simulink model "PUMA_fuzzy_t1"  (Simulink 8.9)
settings: Solver=ode15s  StartTime=0  StopTime=5  MaxStep=0.02  RelTol=1e-3  EnableMultiTasking=on
undefined symbols (not defined in the file or in its folder): sfunxyz
libraries: aerolibutil x17, simulink x4, fuzblock x3
(part 2 of 3)

== system PUMA_fuzzy_t1/3-Link PUMA Robot-Block /A matrix/a22 generator/I5 ==
  AI5 actual I5 : Constant  Value=0.372
  Sum4 : Sum  Inputs=|++
  UI5 uncertainty added to I5 +- 0.05 max : Constant  Value=UI5
  I5 : Outport
  wires:
  AI5 actual I5/1 -> Sum4/1
  UI5 uncertainty added to I5 +- 0.05 max/1 -> Sum4/2
  Sum4/1 -> I5/1

== system PUMA_fuzzy_t1/3-Link PUMA Robot-Block /A matrix/a22 generator/I6 ==
  AI6 actual I6 : Constant  Value=0.333
  Sum4 : Sum  Inputs=|++
  UI6 uncertainty added to I6 +- 0.05 max : Constant  Value=UI6
  I6 : Outport
  wires:
  AI6 actual I6/1 -> Sum4/1
  UI6 uncertainty added to I6 +- 0.05 max/1 -> Sum4/2
  Sum4/1 -> I6/1

== system PUMA_fuzzy_t1/3-Link PUMA Robot-Block /A matrix/a22 generator/Im2 ==
  AIm2 actual Im2 : Constant  Value=4.71
  Sum4 : Sum  Inputs=|++
  UIm2 uncertainty added to Im2 +- 0.54 max : Constant  Value=UIm2
  Im2 : Outport
  wires:
  AIm2 actual Im2/1 -> Sum4/1
  UIm2 uncertainty added to Im2 +- 0.54 max/1 -> Sum4/2
  Sum4/1 -> Im2/1

== system PUMA_fuzzy_t1/3-Link PUMA Robot-Block /A matrix/a23 generator/I12 ==
  AI12 actual I12 : Constant  Value=-0.011
  Sum4 : Sum  Inputs=|++
  UI12 uncertainty added to I12 +- 0.0011 max : Constant  Value=UI12
  I12 : Outport
  wires:
  AI12 actual I12/1 -> Sum4/1
  UI12 uncertainty added to I12 +- 0.0011 max/1 -> Sum4/2
  Sum4/1 -> I12/1

== system PUMA_fuzzy_t1/3-Link PUMA Robot-Block /A matrix/a23 generator/I15 ==
  AI15 actual I15 : Constant  Value=0.00125
  Sum4 : Sum  Inputs=|++
  UI15 uncertainty added to I15 +- 0.0003 max : Constant  Value=UI15
  I15 : Outport
  wires:
  AI15 actual I15/1 -> Sum4/1
  UI15 uncertainty added to I15 +- 0.0003 max/1 -> Sum4/2
  Sum4/1 -> I15/1

== system PUMA_fuzzy_t1/3-Link PUMA Robot-Block /A matrix/a23 generator/I16 ==
  AI16 actual I16 : Constant  Value=0.00124
  Sum4 : Sum  Inputs=|++
  UI16 uncertainty added to I16 +- 0.0003 max : Constant  Value=UI16
  I16 : Outport
  wires:
  AI16 actual I16/1 -> Sum4/1
  UI16 uncertainty added to I16 +- 0.0003 max/1 -> Sum4/2
  Sum4/1 -> I16/1

== system PUMA_fuzzy_t1/3-Link PUMA Robot-Block /A matrix/a23 generator/I5 ==
  AI5 actual I5 : Constant  Value=0.372
  Sum4 : Sum  Inputs=|++
  UI5 uncertainty added to I5 +- 0.05 max : Constant  Value=UI5
  I5 : Outport
  wires:
  AI5 actual I5/1 -> Sum4/1
  UI5 uncertainty added to I5 +- 0.05 max/1 -> Sum4/2
  Sum4/1 -> I5/1

== system PUMA_fuzzy_t1/3-Link PUMA Robot-Block /A matrix/a23 generator/I6 ==
  AI6 actual I6 : Constant  Value=0.333
  Sum4 : Sum  Inputs=|++
  UI6 uncertainty added to I6 +- 0.05 max : Constant  Value=UI6
  I6 : Outport
  wires:
  AI6 actual I6/1 -> Sum4/1
  UI6 uncertainty added to I6 +- 0.05 max/1 -> Sum4/2
  Sum4/1 -> I6/1

== system PUMA_fuzzy_t1/3-Link PUMA Robot-Block /A matrix/a33 generator/I15 ==
  AI15 actual I15 : Constant  Value=0.00125
  Sum4 : Sum  Inputs=|++
  UI15 uncertainty added to I15 +- 0.0003 max : Constant  Value=UI15
  I15 : Outport
  wires:
  AI15 actual I15/1 -> Sum4/1
  UI15 uncertainty added to I15 +- 0.0003 max/1 -> Sum4/2
  Sum4/1 -> I15/1

== system PUMA_fuzzy_t1/3-Link PUMA Robot-Block /A matrix/a33 generator/I6 ==
  AI6 actual I6 : Constant  Value=0.333
  Sum4 : Sum  Inputs=|++
  UI6 uncertainty added to I6 +- 0.05 max : Constant  Value=UI6
  I6 : Outport
  wires:
  AI6 actual I6/1 -> Sum4/1
  UI6 uncertainty added to I6 +- 0.05 max/1 -> Sum4/2
  Sum4/1 -> I6/1

== system PUMA_fuzzy_t1/3-Link PUMA Robot-Block /A matrix/a33 generator/Im3 ==
  AIm3 actual Im3 : Constant  Value=0.827
  Sum4 : Sum  Inputs=|++
  UIm3 uncertainty added to Im3 +- 0.093 max : Constant  Value=UIm3
  Im3 : Outport
  wires:
  AIm3 actual Im3/1 -> Sum4/1
  UIm3 uncertainty added to Im3 +- 0.093 max/1 -> Sum4/2
  Sum4/1 -> Im3/1

== system PUMA_fuzzy_t1/3-Link PUMA Robot-Block /A matrix/a35 generator/I15 ==
  AI15 actual I15 : Constant  Value=0.00125
  Sum4 : Sum  Inputs=|++
  UI15 uncertainty added to I15 +- 0.0003 max : Constant  Value=UI15
  I15 : Outport
  wires:
  AI15 actual I15/1 -> Sum4/1
  UI15 uncertainty added to I15 +- 0.0003 max/1 -> Sum4/2
  Sum4/1 -> I15/1

== system PUMA_fuzzy_t1/3-Link PUMA Robot-Block /A matrix/a35 generator/I17 ==
  AI17 actual I17 : Constant  Value=0.000642
  Sum4 : Sum  Inputs=|++
  UI17 uncertainty added to I17 +- 0.0003 max : Constant  Value=UI17
  I17 : Outport
  wires:
  AI17 actual I17/1 -> Sum4/1
  UI17 uncertainty added to I17 +- 0.0003 max/1 -> Sum4/2
  Sum4/1 -> I17/1

== system PUMA_fuzzy_t1/3-Link PUMA Robot-Block /A matrix/a44 generator/I14 ==
  AI14 actual I14 : Constant  Value=0.00164
  Sum4 : Sum  Inputs=|++
  UI14 uncertainty added to I14 +- 0.0009 max : Constant  Value=UI14
  I14 : Outport
  wires:
  AI14 actual I14/1 -> Sum4/1
  UI14 uncertainty added to I14 +- 0.0009 max/1 -> Sum4/2
  Sum4/1 -> I14/1

== system PUMA_fuzzy_t1/3-Link PUMA Robot-Block /A matrix/a44 generator/Im4 ==
  AIm4 actual Im4 : Constant  Value=0.2
  Sum4 : Sum  Inputs=|++
  UIm4 uncertainty added to Im4 +- 0.54 max : Constant  Value=UIm4
  Im4 : Outport
  wires:
  AIm4 actual Im4/1 -> Sum4/1
  UIm4 uncertainty added to Im4 +- 0.54 max/1 -> Sum4/2
  Sum4/1 -> Im4/1

== system PUMA_fuzzy_t1/3-Link PUMA Robot-Block /A matrix/a55 generator/I17 ==
  AI17 actual I17 : Constant  Value=0.000642
  Sum4 : Sum  Inputs=|++
  UI17 uncertainty added to I17 +- 0.0003 max : Constant  Value=UI17
  I17 : Outport
  wires:
  AI17 actual I17/1 -> Sum4/1
  UI17 uncertainty added to I17 +- 0.0003 max/1 -> Sum4/2
  Sum4/1 -> I17/1

== system PUMA_fuzzy_t1/3-Link PUMA Robot-Block /A matrix/a55 generator/Im5 ==
  AIm5 actual Im5 : Constant  Value=0.179
  Sum4 : Sum  Inputs=|++
  UIm5 uncertainty added to Im5 +- 0.014 max : Constant  Value=UIm5
  Im5 : Outport
  wires:
  AIm5 actual Im5/1 -> Sum4/1
  UIm5 uncertainty added to Im5 +- 0.014 max/1 -> Sum4/2
  Sum4/1 -> Im5/1

== system PUMA_fuzzy_t1/3-Link PUMA Robot-Block /A matrix/a66 generator/I23 ==
  AI23 actual I23 : Constant  Value=0.00004
  Sum4 : Sum  Inputs=|++
  UI23 uncertainty added to I23 +- 0.00002 max : Constant  Value=UI23
  I23 : Outport
  wires:
  AI23 actual I23/1 -> Sum4/1
  UI23 uncertainty added to I23 +- 0.00002 max/1 -> Sum4/2
  Sum4/1 -> I23/1

== system PUMA_fuzzy_t1/3-Link PUMA Robot-Block /A matrix/a66 generator/Im6 ==
  AIm6 actual Im6 : Constant  Value=0.193
  Sum4 : Sum  Inputs=|++
  UIm6 uncertainty added to Im6 +- 0.54 max : Constant  Value=UIm6
  Im6 : Outport
  wires:
  AIm6 actual Im6/1 -> Sum4/1
  UIm6 uncertainty added to Im6 +- 0.54 max/1 -> Sum4/2
  Sum4/1 -> Im6/1

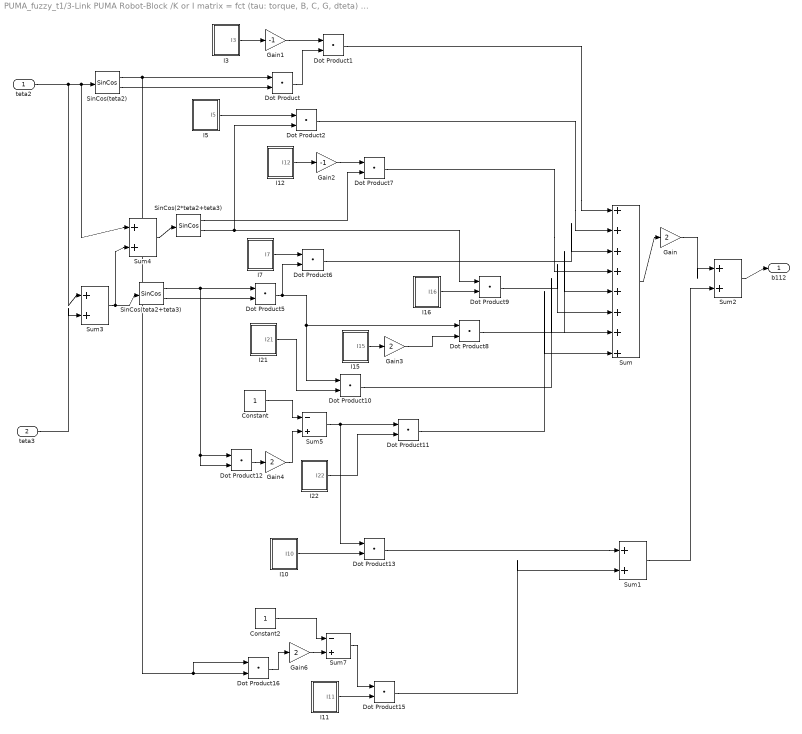
== system PUMA_fuzzy_t1/3-Link PUMA Robot-Block /K or I matrix = fct (tau: torque, B, C, G, dteta) /B matrix/b112 ==
  teta2 : Inport
  teta3 : Inport  Port=2
  Constant : Constant
  Constant2 : Constant
  Dot Product{,1..2,5..13,15..16} (14 alike) : DotProduct  InputSameDT=on  OutDataTypeStr=Inherit: Inherit via internal rule
  Gain{,3..4,6} (4 alike) : Gain  Gain=2
  Gain1 : Gain  Gain=-1
  Gain2 : Gain  Gain=-1
  I10 : Subsystem
  I11 : Subsystem
  I12 : Subsystem
  I15 : Subsystem
  I16 : Subsystem
  I21 : Subsystem
  I22 : Subsystem
  I3 : Subsystem
  I5 : Subsystem
  I7 : Subsystem
  SinCos(2*teta2+teta3) : aerolibutil/SinCos
      settings: SourceProductName=Aerospace Blockset  SourceProductBaseCode=AE
  SinCos(teta2) : aerolibutil/SinCos
      settings: SourceProductName=Aerospace Blockset  SourceProductBaseCode=AE
  SinCos(teta2+teta3) : aerolibutil/SinCos
      settings: SourceProductName=Aerospace Blockset  SourceProductBaseCode=AE
  Sum : Sum  Inputs=|++++++++
  Sum{1..4} (4 alike) : Sum  Inputs=|++
  Sum5 : Sum  Inputs=|-+
  Sum7 : Sum  Inputs=|-+
  b112 : Outport
  wires:
  Sum/1 -> Gain/1
  Gain/1 -> Sum2/1
  Sum1/1 -> Sum2/2
  Sum2/1 -> b112/1
  teta2/1 -> Sum4/1, SinCos(teta2)/1, Sum3/1
  teta3/1 -> Sum3/2
  SinCos(teta2)/1 -> Dot Product/1, Dot Product16/2, Dot Product16/1
  SinCos(teta2)/2 -> Dot Product/2
  Sum3/1 -> SinCos(teta2+teta3)/1, Sum4/2
  I3/1(I3) -> Gain1/1
  Gain1/1 -> Dot Product1/1
  Dot Product/1 -> Dot Product1/2
  Dot Product1/1 -> Sum/1
  Dot Product2/1 -> Sum/2
  I7/1(I7) -> Dot Product6/1
  Dot Product5/1 -> Dot Product6/2, Dot Product8/1, Dot Product10/1
  SinCos(teta2+teta3)/1 -> Dot Product5/1, Dot Product12/1, Dot Product12/2
  SinCos(teta2+teta3)/2 -> Dot Product5/2
  Dot Product6/1 -> Sum/3
  I12/1(I12) -> Gain2/1
  Sum4/1 -> SinCos(2*teta2+teta3)/1
  Gain2/1 -> Dot Product7/1
  SinCos(2*teta2+teta3)/1 -> Dot Product7/2
  Dot Product7/1 -> Sum/4
  I15/1(I15) -> Gain3/1
  Gain3/1 -> Dot Product8/2
  Dot Product8/1 -> Sum/5
  SinCos(2*teta2+teta3)/2 -> Dot Product9/1, Dot Product2/2
  I16/1(I16) -> Dot Product9/2
  Dot Product9/1 -> Sum/6
  I21/1(I21) -> Dot Product10/2
  Dot Product10/1 -> Sum/7
  I22/1(I22) -> Dot Product11/2
  Dot Product12/1 -> Gain4/1
  Constant/1 -> Sum5/1
  Gain4/1 -> Sum5/2
  Sum5/1 -> Dot Product13/1, Dot Product11/1
  Dot Product11/1 -> Sum/8
  I10/1(I10) -> Dot Product13/2
  I11/1(I11) -> Dot Product15/2
  Dot Product16/1 -> Gain6/1
  Constant2/1 -> Sum7/1
  Gain6/1 -> Sum7/2
  Sum7/1 -> Dot Product15/1
  Dot Product13/1 -> Sum1/1
  Dot Product15/1 -> Sum1/2
  I5/1(I5) -> Dot Product2/1

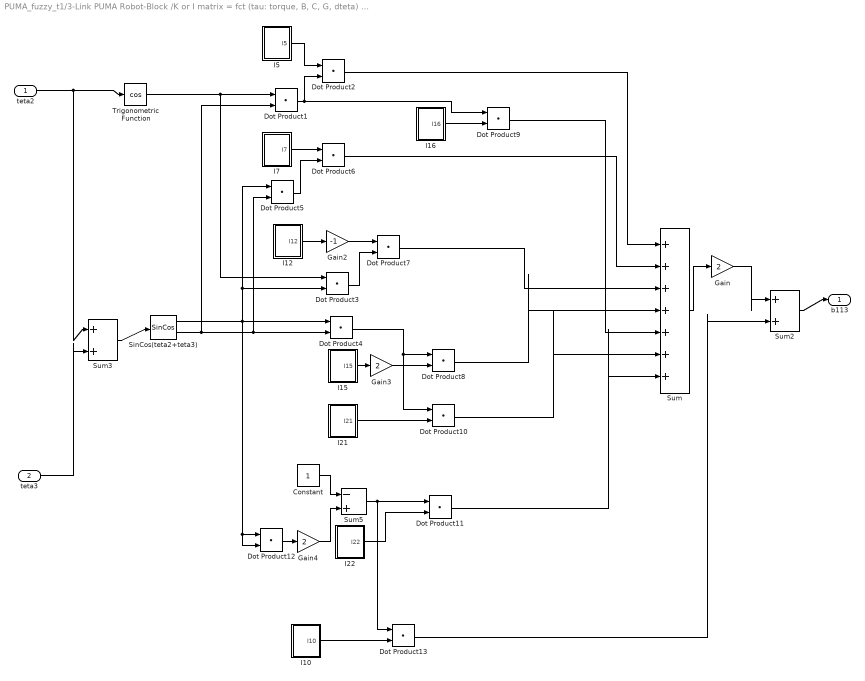
== system PUMA_fuzzy_t1/3-Link PUMA Robot-Block /K or I matrix = fct (tau: torque, B, C, G, dteta) /B matrix/b113 ==
  teta2 : Inport
  teta3 : Inport  Port=2
  Constant : Constant
  Dot Product{1..13} (13 alike) : DotProduct  InputSameDT=on  OutDataTypeStr=Inherit: Inherit via internal rule
  Gain : Gain  Gain=2
  Gain2 : Gain  Gain=-1
  Gain3 : Gain  Gain=2
  Gain4 : Gain  Gain=2
  I10 : Subsystem
  I12 : Subsystem
  I15 : Subsystem
  I16 : Subsystem
  I21 : Subsystem
  I22 : Subsystem
  I5 : Subsystem
  I7 : Subsystem
  SinCos(teta2+teta3) : aerolibutil/SinCos
      settings: SourceProductName=Aerospace Blockset  SourceProductBaseCode=AE
  Sum : Sum  Inputs=|+++++++
  Sum2 : Sum  Inputs=|++
  Sum3 : Sum  Inputs=|++
  Sum5 : Sum  Inputs=|-+
  Trigonometric Function : Trigonometry  Operator=cos
  b113 : Outport
  wires:
  Sum/1 -> Gain/1
  Gain/1 -> Sum2/1
  Sum2/1 -> b113/1
  teta2/1 -> Sum3/1, Trigonometric Function/1
  teta3/1 -> Sum3/2
  Sum3/1 -> SinCos(teta2+teta3)/1
  I7/1(I7) -> Dot Product6/1
  Dot Product5/1 -> Dot Product6/2
  SinCos(teta2+teta3)/1 -> Dot Product5/1, Dot Product3/2, Dot Product4/1, Dot Product12/1, Dot Product12/2
  SinCos(teta2+teta3)/2 -> Dot Product1/2, Dot Product5/2, Dot Product4/2
  I12/1(I12) -> Gain2/1
  Gain2/1 -> Dot Product7/1
  I15/1(I15) -> Gain3/1
  Gain3/1 -> Dot Product8/2
  I16/1(I16) -> Dot Product9/2
  I21/1(I21) -> Dot Product10/2
  I22/1(I22) -> Dot Product11/2
  Dot Product12/1 -> Gain4/1
  Constant/1 -> Sum5/1
  Gain4/1 -> Sum5/2
  Sum5/1 -> Dot Product13/1, Dot Product11/1
  I10/1(I10) -> Dot Product13/2
  I5/1(I5) -> Dot Product2/1
  Dot Product1/1 -> Dot Product2/2, Dot Product9/1
  Trigonometric Function/1 -> Dot Product1/1, Dot Product3/1
  Dot Product3/1 -> Dot Product7/2
  Dot Product4/1 -> Dot Product8/1, Dot Product10/1
  Dot Product13/1 -> Sum2/2
  Dot Product2/1 -> Sum/1
  Dot Product6/1 -> Sum/2
  Dot Product7/1 -> Sum/3
  Dot Product8/1 -> Sum/4
  Dot Product9/1 -> Sum/5
  Dot Product10/1 -> Sum/6
  Dot Product11/1 -> Sum/7

== system PUMA_fuzzy_t1/3-Link PUMA Robot-Block /K or I matrix = fct (tau: torque, B, C, G, dteta) /B matrix/b115 ==
  teta2 : Inport
  teta3 : Inport  Port=2
  Dot Product{,1..5} (6 alike) : DotProduct  InputSameDT=on  OutDataTypeStr=Inherit: Inherit via internal rule
  Gain : Gain  Gain=2
  Gain1 : Gain  Gain=-1
  I15 : Subsystem
  I16 : Subsystem
  I22 : Subsystem
  SinCos(teta2+teta3) : aerolibutil/SinCos
      settings: SourceProductName=Aerospace Blockset  SourceProductBaseCode=AE
  Sum2 : Sum  Inputs=|++++
  Sum3 : Sum  Inputs=|++
  Trigonometric Function : Trigonometry  Operator=cos
  b115 : Outport
  wires:
  teta2/1 -> Sum3/1, Trigonometric Function/1
  teta3/1 -> Sum3/2
  Sum3/1 -> SinCos(teta2+teta3)/1
  SinCos(teta2+teta3)/1 -> Dot Product/1
  SinCos(teta2+teta3)/2 -> Dot Product/2, Dot Product3/1, Dot Product5/1, Dot Product5/2
  Dot Product/1 -> Gain1/1, Dot Product1/1
  I15/1(I15) -> Dot Product1/2
  I16/1(I16) -> Dot Product2/2
  Dot Product3/1 -> Dot Product2/1
  Trigonometric Function/1 -> Dot Product3/2
  Sum2/1 -> Gain/1
  Gain/1 -> b115/1
  I22/1(I22) -> Dot Product4/2
  Dot Product5/1 -> Dot Product4/1
  Gain1/1 -> Sum2/1
  Dot Product1/1 -> Sum2/2
  Dot Product2/1 -> Sum2/3
  Dot Product4/1 -> Sum2/4

== system PUMA_fuzzy_t1/3-Link PUMA Robot-Block /K or I matrix = fct (tau: torque, B, C, G, dteta) /B matrix/b123 ==
  teta2 : Inport
  teta3 : Inport  Port=2
  Dot Product : DotProduct  InputSameDT=on  OutDataTypeStr=Inherit: Inherit via internal rule
  Dot Product1 : DotProduct  InputSameDT=on  OutDataTypeStr=Inherit: Inherit via internal rule
  Dot Product2 : DotProduct  InputSameDT=on  OutDataTypeStr=Inherit: Inherit via internal rule
  Gain : Gain  Gain=2
  Gain1 : Gain  Gain=-1
  I13 : Subsystem
  I18 : Subsystem
  I8 : Subsystem
  SinCos(teta2+teta3) : aerolibutil/SinCos
      settings: SourceProductName=Aerospace Blockset  SourceProductBaseCode=AE
  Sum2 : Sum  Inputs=|+++
  Sum3 : Sum  Inputs=|++
  b123 : Outport
  wires:
  teta2/1 -> Sum3/1
  teta3/1 -> Sum3/2
  Sum3/1 -> SinCos(teta2+teta3)/1
  Dot Product/1 -> Gain1/1
  Sum2/1 -> Gain/1
  Gain/1 -> b123/1
  SinCos(teta2+teta3)/1 -> Dot Product/2, Dot Product2/1
  I8/1(I8) -> Dot Product/1
  SinCos(teta2+teta3)/2 -> Dot Product1/1
  I13/1(I13) -> Dot Product1/2
  I18/1(I18) -> Dot Product2/2
  Gain1/1 -> Sum2/1
  Dot Product1/1 -> Sum2/2
  Dot Product2/1 -> Sum2/3

== system PUMA_fuzzy_t1/3-Link PUMA Robot-Block /K or I matrix = fct (tau: torque, B, C, G, dteta) /B matrix/b214 ==
  teta2 : Inport
  teta3 : Inport  Port=2
  Dot Product1 : DotProduct  InputSameDT=on  OutDataTypeStr=Inherit: Inherit via internal rule
  Dot Product2 : DotProduct  InputSameDT=on  OutDataTypeStr=Inherit: Inherit via internal rule
  Dot Product3 : DotProduct  InputSameDT=on  OutDataTypeStr=Inherit: Inherit via internal rule
  I14 : Subsystem
  I19 : Subsystem
  I20 : Subsystem
  Sum2 : Sum  Inputs=|+++
  Sum3 : Sum  Inputs=|++
  sin(teta2+teta3) : Trigonometry
  b214 : Outport
  wires:
  teta2/1 -> Sum3/1
  teta3/1 -> Sum3/2
  Sum3/1 -> sin(teta2+teta3)/1
  Sum2/1 -> b214/1
  I14/1(I14) -> Dot Product3/1
  sin(teta2+teta3)/1 -> Dot Product3/2, Dot Product1/1, Dot Product2/1
  I19/1(I19) -> Dot Product1/2
  I20/1(I20) -> Dot Product2/2
  Dot Product3/1 -> Sum2/1
  Dot Product1/1 -> Sum2/2
  Dot Product2/1 -> Sum2/3

== system PUMA_fuzzy_t1/3-Link PUMA Robot-Block /K or I matrix = fct (tau: torque, B, C, G, dteta) /B matrix/b223 ==
  teta3 : Inport
  Dot Product1 : DotProduct  InputSameDT=on  OutDataTypeStr=Inherit: Inherit via internal rule
  Dot Product2 : DotProduct  InputSameDT=on  OutDataTypeStr=Inherit: Inherit via internal rule
  Dot Product3 : DotProduct  InputSameDT=on  OutDataTypeStr=Inherit: Inherit via internal rule
  Gain : Gain  Gain=2
  I12 : Subsystem
  I16 : Subsystem
  I5 : Subsystem
  SinCos(teta2+teta3) : aerolibutil/SinCos
      settings: SourceProductName=Aerospace Blockset  SourceProductBaseCode=AE
  Sum2 : Sum  Inputs=|-++
  b223 : Outport
  wires:
  teta3/1 -> SinCos(teta2+teta3)/1
  Dot Product3/1 -> Sum2/1
  Dot Product1/1 -> Sum2/2
  Dot Product2/1 -> Sum2/3
  Sum2/1 -> Gain/1
  Gain/1 -> b223/1
  I12/1(I12) -> Dot Product3/1
  I5/1(I5) -> Dot Product1/2
  I16/1(I16) -> Dot Product2/2
  SinCos(teta2+teta3)/2 -> Dot Product2/1, Dot Product1/1
  SinCos(teta2+teta3)/1 -> Dot Product3/2

== system PUMA_fuzzy_t1/3-Link PUMA Robot-Block /K or I matrix = fct (tau: torque, B, C, G, dteta) /B matrix/b225 ==
  teta3 : Inport
  Dot Product2 : DotProduct  InputSameDT=on  OutDataTypeStr=Inherit: Inherit via internal rule
  Gain : Gain  Gain=2
  I16 : Subsystem
  I22 : Subsystem
  Sum2 : Sum  Inputs=|++
  cos(teta3) : Trigonometry  Operator=cos
  b225 : Outport
  wires:
  teta3/1 -> cos(teta3)/1
  Sum2/1 -> Gain/1
  Gain/1 -> b225/1
  Dot Product2/1 -> Sum2/1
  I22/1(I22) -> Sum2/2
  I16/1(I16) -> Dot Product2/1
  cos(teta3)/1 -> Dot Product2/2

== system PUMA_fuzzy_t1/3-Link PUMA Robot-Block /K or I matrix = fct (tau: torque, B, C, G, dteta) /B matrix/b235 ==
  teta3 : Inport
  Dot Product2 : DotProduct  InputSameDT=on  OutDataTypeStr=Inherit: Inherit via internal rule
  Gain : Gain  Gain=2
  I16 : Subsystem
  I22 : Subsystem
  Sum2 : Sum  Inputs=|++
  cos(teta3) : Trigonometry  Operator=cos
  b235 : Outport
  wires:
  teta3/1 -> cos(teta3)/1
  Sum2/1 -> Gain/1
  Gain/1 -> b235/1
  Dot Product2/1 -> Sum2/1
  I22/1(I22) -> Sum2/2
  I16/1(I16) -> Dot Product2/1
  cos(teta3)/1 -> Dot Product2/2

== system PUMA_fuzzy_t1/3-Link PUMA Robot-Block /K or I matrix = fct (tau: torque, B, C, G, dteta) /B matrix/b314 ==
  teta2 : Inport
  teta3 : Inport  Port=2
  Dot Product1 : DotProduct  InputSameDT=on  OutDataTypeStr=Inherit: Inherit via internal rule
  Dot Product2 : DotProduct  InputSameDT=on  OutDataTypeStr=Inherit: Inherit via internal rule
  Dot Product3 : DotProduct  InputSameDT=on  OutDataTypeStr=Inherit: Inherit via internal rule
  I14 : Subsystem
  I19 : Subsystem
  I20 : Subsystem
  Sum2 : Sum  Inputs=|+++
  Sum3 : Sum  Inputs=|++
  sin(teta2+teta3) : Trigonometry
  b314 : Outport
  wires:
  teta2/1 -> Sum3/1
  teta3/1 -> Sum3/2
  Sum3/1 -> sin(teta2+teta3)/1
  Sum2/1 -> b314/1
  I14/1(I14) -> Dot Product3/1
  sin(teta2+teta3)/1 -> Dot Product3/2, Dot Product1/1, Dot Product2/1
  I19/1(I19) -> Dot Product1/2
  I20/1(I20) -> Dot Product2/2
  Dot Product3/1 -> Sum2/1
  Dot Product1/1 -> Sum2/2
  Dot Product2/1 -> Sum2/3

== system PUMA_fuzzy_t1/3-Link PUMA Robot-Block /K or I matrix = fct (tau: torque, B, C, G, dteta) /B matrix/b412 ==
  teta2 : Inport
  teta3 : Inport  Port=2
  Dot Product1 : DotProduct  InputSameDT=on  OutDataTypeStr=Inherit: Inherit via internal rule
  Dot Product2 : DotProduct  InputSameDT=on  OutDataTypeStr=Inherit: Inherit via internal rule
  Dot Product3 : DotProduct  InputSameDT=on  OutDataTypeStr=Inherit: Inherit via internal rule
  Gain : Gain  Gain=-1
  I14 : Subsystem
  I19 : Subsystem
  I20 : Subsystem
  Sum2 : Sum  Inputs=|+++
  Sum3 : Sum  Inputs=|++
  sin(teta2+teta3) : Trigonometry
  b412 : Outport
  wires:
  teta2/1 -> Sum3/1
  teta3/1 -> Sum3/2
  Sum3/1 -> sin(teta2+teta3)/1
  I14/1(I14) -> Dot Product3/1
  sin(teta2+teta3)/1 -> Dot Product3/2, Dot Product1/1, Dot Product2/1
  I19/1(I19) -> Dot Product1/2
  I20/1(I20) -> Dot Product2/2
  Dot Product3/1 -> Sum2/1
  Dot Product1/1 -> Sum2/2
  Dot Product2/1 -> Sum2/3
  Sum2/1 -> Gain/1
  Gain/1 -> b412/1

== system PUMA_fuzzy_t1/3-Link PUMA Robot-Block /K or I matrix = fct (tau: torque, B, C, G, dteta) /B matrix/b413 ==
  teta2 : Inport
  teta3 : Inport  Port=2
  Dot Product1 : DotProduct  InputSameDT=on  OutDataTypeStr=Inherit: Inherit via internal rule
  Dot Product2 : DotProduct  InputSameDT=on  OutDataTypeStr=Inherit: Inherit via internal rule
  Dot Product3 : DotProduct  InputSameDT=on  OutDataTypeStr=Inherit: Inherit via internal rule
  Gain : Gain  Gain=-1
  I14 : Subsystem
  I19 : Subsystem
  I20 : Subsystem
  Sum2 : Sum  Inputs=|+++
  Sum3 : Sum  Inputs=|++
  sin(teta2+teta3) : Trigonometry
  b413 : Outport
  wires:
  teta2/1 -> Sum3/1
  teta3/1 -> Sum3/2
  Sum3/1 -> sin(teta2+teta3)/1
  I14/1(I14) -> Dot Product3/1
  sin(teta2+teta3)/1 -> Dot Product3/2, Dot Product1/1, Dot Product2/1
  I19/1(I19) -> Dot Product1/2
  I20/1(I20) -> Dot Product2/2
  Dot Product3/1 -> Sum2/1
  Dot Product1/1 -> Sum2/2
  Dot Product2/1 -> Sum2/3
  Sum2/1 -> Gain/1
  Gain/1 -> b413/1

== system PUMA_fuzzy_t1/3-Link PUMA Robot-Block /K or I matrix = fct (tau: torque, B, C, G, dteta) /B matrix/b415 ==
  teta2 : Inport
  teta3 : Inport  Port=2
  Dot Product2 : DotProduct  InputSameDT=on  OutDataTypeStr=Inherit: Inherit via internal rule
  Dot Product3 : DotProduct  InputSameDT=on  OutDataTypeStr=Inherit: Inherit via internal rule
  Gain : Gain  Gain=-1
  I17 : Subsystem
  I20 : Subsystem
  Sum2 : Sum  Inputs=|++
  Sum3 : Sum  Inputs=|++
  sin(teta2+teta3) : Trigonometry
  b415 : Outport
  wires:
  teta2/1 -> Sum3/1
  teta3/1 -> Sum3/2
  Sum3/1 -> sin(teta2+teta3)/1
  sin(teta2+teta3)/1 -> Dot Product3/2, Dot Product2/1
  I20/1(I20) -> Dot Product2/2
  Dot Product3/1 -> Sum2/1
  I17/1(I17) -> Dot Product3/1
  Dot Product2/1 -> Sum2/2
  Sum2/1 -> Gain/1
  Gain/1 -> b415/1

== system PUMA_fuzzy_t1/3-Link PUMA Robot-Block /K or I matrix = fct (tau: torque, B, C, G, dteta) /B matrix/b514 ==
  teta2 : Inport
  teta3 : Inport  Port=2
  Dot Product2 : DotProduct  InputSameDT=on  OutDataTypeStr=Inherit: Inherit via internal rule
  Dot Product3 : DotProduct  InputSameDT=on  OutDataTypeStr=Inherit: Inherit via internal rule
  I17 : Subsystem
  I20 : Subsystem
  Sum2 : Sum  Inputs=|++
  Sum3 : Sum  Inputs=|++
  sin(teta2+teta3) : Trigonometry
  b514 : Outport
  wires:
  teta2/1 -> Sum3/1
  teta3/1 -> Sum3/2
  Sum3/1 -> sin(teta2+teta3)/1
  sin(teta2+teta3)/1 -> Dot Product3/2, Dot Product2/1
  I20/1(I20) -> Dot Product2/2
  Dot Product3/1 -> Sum2/1
  I17/1(I17) -> Dot Product3/1
  Dot Product2/1 -> Sum2/2
  Sum2/1 -> b514/1

== system PUMA_fuzzy_t1/3-Link PUMA Robot-Block /K or I matrix = fct (tau: torque, B, C, G, dteta) /C matrix/c12 ==
  teta3 : Inport
  teta2 : Inport  Port=2
  Dot Product{1..5} (5 alike) : DotProduct  InputSameDT=on  OutDataTypeStr=Inherit: Inherit via internal rule
  I13 : Subsystem
  I18 : Subsystem
  I4 : Subsystem
  I8 : Subsystem
  I9 : Subsystem
  SinCos(teta2) : aerolibutil/SinCos
      settings: SourceProductName=Aerospace Blockset  SourceProductBaseCode=AE
  SinCos(teta2+teta3) : aerolibutil/SinCos
      settings: SourceProductName=Aerospace Blockset  SourceProductBaseCode=AE
  Sum1 : Sum  Inputs=|++
  Sum2 : Sum  Inputs=|+--++
  c12 : Outport
  wires:
  Dot Product3/1 -> Sum2/1
  Dot Product1/1 -> Sum2/2
  Dot Product2/1 -> Sum2/3
  Sum2/1 -> c12/1
  teta2/1 -> Sum1/1, SinCos(teta2)/1
  teta3/1 -> Sum1/2
  Sum1/1 -> SinCos(teta2+teta3)/1
  Dot Product4/1 -> Sum2/4
  Dot Product5/1 -> Sum2/5
  I4/1(I4) -> Dot Product3/1
  SinCos(teta2)/2 -> Dot Product3/2
  I8/1(I8) -> Dot Product1/1
  SinCos(teta2+teta3)/1 -> Dot Product1/2, Dot Product5/1
  SinCos(teta2)/1 -> Dot Product2/1
  I9/1(I9) -> Dot Product2/2
  SinCos(teta2+teta3)/2 -> Dot Product4/1
  I13/1(I13) -> Dot Product4/2
  I18/1(I18) -> Dot Product5/2

== system PUMA_fuzzy_t1/3-Link PUMA Robot-Block /K or I matrix = fct (tau: torque, B, C, G, dteta) /C matrix/c13 ==
  teta2 : Inport
  teta3 : Inport  Port=2
  Dot Product : DotProduct  InputSameDT=on  OutDataTypeStr=Inherit: Inherit via internal rule
  Dot Product1 : DotProduct  InputSameDT=on  OutDataTypeStr=Inherit: Inherit via internal rule
  Dot Product2 : DotProduct  InputSameDT=on  OutDataTypeStr=Inherit: Inherit via internal rule
  Gain1 : Gain  Gain=-1
  I13 : Subsystem
  I18 : Subsystem
  I8 : Subsystem
  SinCos(teta2+teta3) : aerolibutil/SinCos
      settings: SourceProductName=Aerospace Blockset  SourceProductBaseCode=AE
  Sum2 : Sum  Inputs=|+++
  Sum3 : Sum  Inputs=|++
  c13 : Outport
  wires:
  teta2/1 -> Sum3/1
  teta3/1 -> Sum3/2
  Sum3/1 -> SinCos(teta2+teta3)/1
  Dot Product/1 -> Gain1/1
  SinCos(teta2+teta3)/1 -> Dot Product/2, Dot Product2/1
  I8/1(I8) -> Dot Product/1
  SinCos(teta2+teta3)/2 -> Dot Product1/1
  I13/1(I13) -> Dot Product1/2
  I18/1(I18) -> Dot Product2/2
  Gain1/1 -> Sum2/1
  Dot Product1/1 -> Sum2/2
  Dot Product2/1 -> Sum2/3
  Sum2/1 -> c13/1

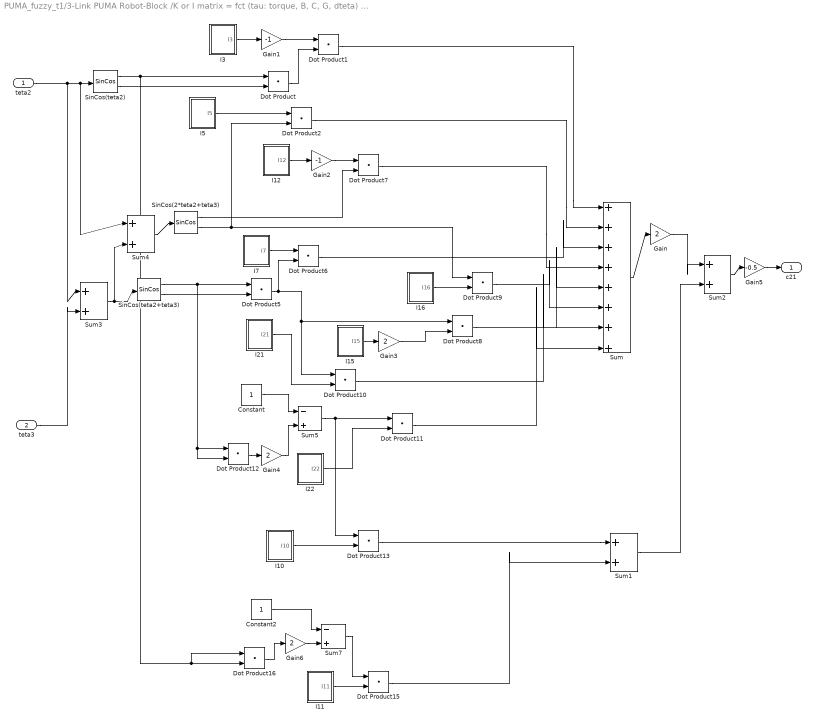
== system PUMA_fuzzy_t1/3-Link PUMA Robot-Block /K or I matrix = fct (tau: torque, B, C, G, dteta) /C matrix/c21 ==
  teta2 : Inport
  teta3 : Inport  Port=2
  Constant : Constant
  Constant2 : Constant
  Dot Product{,1..2,5..13,15..16} (14 alike) : DotProduct  InputSameDT=on  OutDataTypeStr=Inherit: Inherit via internal rule
  Gain{,3..4,6} (4 alike) : Gain  Gain=2
  Gain1 : Gain  Gain=-1
  Gain2 : Gain  Gain=-1
  Gain5 : Gain  Gain=-0.5
  I10 : Subsystem
  I11 : Subsystem
  I12 : Subsystem
  I15 : Subsystem
  I16 : Subsystem
  I21 : Subsystem
  I22 : Subsystem
  I3 : Subsystem
  I5 : Subsystem
  I7 : Subsystem
  SinCos(2*teta2+teta3) : aerolibutil/SinCos
      settings: SourceProductName=Aerospace Blockset  SourceProductBaseCode=AE
  SinCos(teta2) : aerolibutil/SinCos
      settings: SourceProductName=Aerospace Blockset  SourceProductBaseCode=AE
  SinCos(teta2+teta3) : aerolibutil/SinCos
      settings: SourceProductName=Aerospace Blockset  SourceProductBaseCode=AE
  Sum : Sum  Inputs=|++++++++
  Sum{1..4} (4 alike) : Sum  Inputs=|++
  Sum5 : Sum  Inputs=|-+
  Sum7 : Sum  Inputs=|-+
  c21 : Outport
  wires:
  Sum/1 -> Gain/1
  Gain/1 -> Sum2/1
  Sum1/1 -> Sum2/2
  teta2/1 -> Sum4/1, SinCos(teta2)/1, Sum3/1
  teta3/1 -> Sum3/2
  SinCos(teta2)/1 -> Dot Product/1, Dot Product16/2, Dot Product16/1
  SinCos(teta2)/2 -> Dot Product/2
  Sum3/1 -> SinCos(teta2+teta3)/1, Sum4/2
  I3/1(I3) -> Gain1/1
  Gain1/1 -> Dot Product1/1
  Dot Product/1 -> Dot Product1/2
  Dot Product1/1 -> Sum/1
  Dot Product2/1 -> Sum/2
  I7/1(I7) -> Dot Product6/1
  Dot Product5/1 -> Dot Product6/2, Dot Product8/1, Dot Product10/1
  SinCos(teta2+teta3)/1 -> Dot Product5/1, Dot Product12/1, Dot Product12/2
  SinCos(teta2+teta3)/2 -> Dot Product5/2
  Dot Product6/1 -> Sum/3
  I12/1(I12) -> Gain2/1
  Sum4/1 -> SinCos(2*teta2+teta3)/1
  Gain2/1 -> Dot Product7/1
  SinCos(2*teta2+teta3)/1 -> Dot Product7/2
  Dot Product7/1 -> Sum/4
  I15/1(I15) -> Gain3/1
  Gain3/1 -> Dot Product8/2
  Dot Product8/1 -> Sum/5
  SinCos(2*teta2+teta3)/2 -> Dot Product9/1, Dot Product2/2
  I16/1(I16) -> Dot Product9/2
  Dot Product9/1 -> Sum/6
  I21/1(I21) -> Dot Product10/2
  Dot Product10/1 -> Sum/7
  I22/1(I22) -> Dot Product11/2
  Dot Product12/1 -> Gain4/1
  Constant/1 -> Sum5/1
  Gain4/1 -> Sum5/2
  Sum5/1 -> Dot Product13/1, Dot Product11/1
  Dot Product11/1 -> Sum/8
  I10/1(I10) -> Dot Product13/2
  I11/1(I11) -> Dot Product15/2
  Dot Product16/1 -> Gain6/1
  Constant2/1 -> Sum7/1
  Gain6/1 -> Sum7/2
  Sum7/1 -> Dot Product15/1
  Dot Product13/1 -> Sum1/1
  Dot Product15/1 -> Sum1/2
  I5/1(I5) -> Dot Product2/1
  Sum2/1 -> Gain5/1
  Gain5/1 -> c21/1

== system PUMA_fuzzy_t1/3-Link PUMA Robot-Block /K or I matrix = fct (tau: torque, B, C, G, dteta) /C matrix/c23 ==
  teta3 : Inport
  Dot Product1 : DotProduct  InputSameDT=on  OutDataTypeStr=Inherit: Inherit via internal rule
  Dot Product2 : DotProduct  InputSameDT=on  OutDataTypeStr=Inherit: Inherit via internal rule
  Dot Product3 : DotProduct  InputSameDT=on  OutDataTypeStr=Inherit: Inherit via internal rule
  I12 : Subsystem
  I16 : Subsystem
  I5 : Subsystem
  SinCos(teta2+teta3) : aerolibutil/SinCos
      settings: SourceProductName=Aerospace Blockset  SourceProductBaseCode=AE
  Sum2 : Sum  Inputs=|-++
  c23 : Outport
  wires:
  teta3/1 -> SinCos(teta2+teta3)/1
  Dot Product3/1 -> Sum2/1
  Dot Product1/1 -> Sum2/2
  Dot Product2/1 -> Sum2/3
  I12/1(I12) -> Dot Product3/1
  I5/1(I5) -> Dot Product1/2
  I16/1(I16) -> Dot Product2/2
  SinCos(teta2+teta3)/2 -> Dot Product2/1, Dot Product1/1
  SinCos(teta2+teta3)/1 -> Dot Product3/2
  Sum2/1 -> c23/1

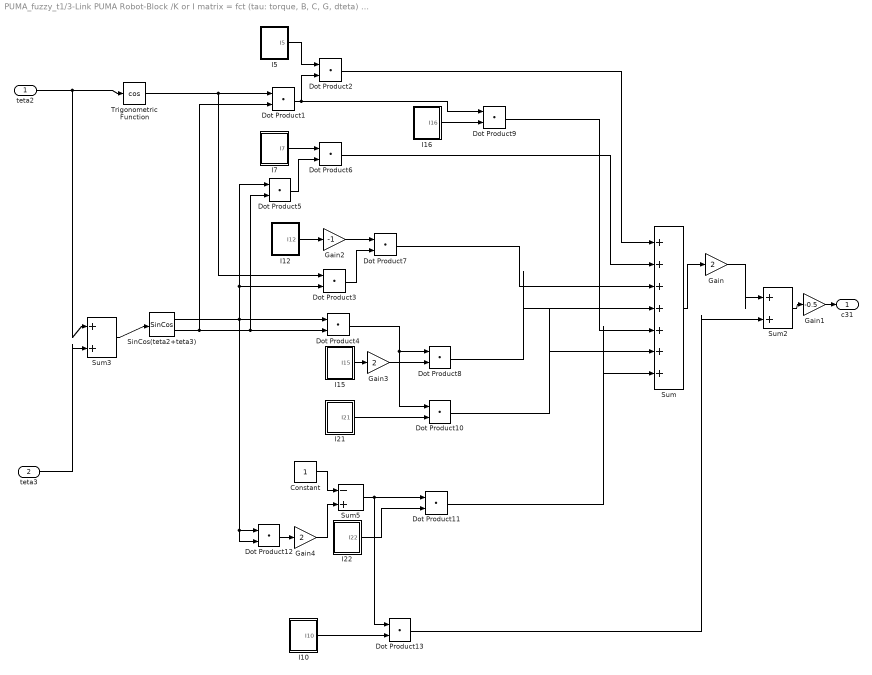
== system PUMA_fuzzy_t1/3-Link PUMA Robot-Block /K or I matrix = fct (tau: torque, B, C, G, dteta) /C matrix/c31 ==
  teta2 : Inport
  teta3 : Inport  Port=2
  Constant : Constant
  Dot Product{1..13} (13 alike) : DotProduct  InputSameDT=on  OutDataTypeStr=Inherit: Inherit via internal rule
  Gain : Gain  Gain=2
  Gain1 : Gain  Gain=-0.5
  Gain2 : Gain  Gain=-1
  Gain3 : Gain  Gain=2
  Gain4 : Gain  Gain=2
  I10 : Subsystem
  I12 : Subsystem
  I15 : Subsystem
  I16 : Subsystem
  I21 : Subsystem
  I22 : Subsystem
  I5 : Subsystem
  I7 : Subsystem
  SinCos(teta2+teta3) : aerolibutil/SinCos
      settings: SourceProductName=Aerospace Blockset  SourceProductBaseCode=AE
  Sum : Sum  Inputs=|+++++++
  Sum2 : Sum  Inputs=|++
  Sum3 : Sum  Inputs=|++
  Sum5 : Sum  Inputs=|-+
  Trigonometric Function : Trigonometry  Operator=cos
  c31 : Outport
  wires:
  Sum/1 -> Gain/1
  Gain/1 -> Sum2/1
  teta2/1 -> Sum3/1, Trigonometric Function/1
  teta3/1 -> Sum3/2
  Sum3/1 -> SinCos(teta2+teta3)/1
  I7/1(I7) -> Dot Product6/1
  Dot Product5/1 -> Dot Product6/2
  SinCos(teta2+teta3)/1 -> Dot Product5/1, Dot Product3/2, Dot Product4/1, Dot Product12/1, Dot Product12/2
  SinCos(teta2+teta3)/2 -> Dot Product1/2, Dot Product5/2, Dot Product4/2
  I12/1(I12) -> Gain2/1
  Gain2/1 -> Dot Product7/1
  I15/1(I15) -> Gain3/1
  Gain3/1 -> Dot Product8/2
  I16/1(I16) -> Dot Product9/2
  I21/1(I21) -> Dot Product10/2
  I22/1(I22) -> Dot Product11/2
  Dot Product12/1 -> Gain4/1
  Constant/1 -> Sum5/1
  Gain4/1 -> Sum5/2
  Sum5/1 -> Dot Product13/1, Dot Product11/1
  I10/1(I10) -> Dot Product13/2
  I5/1(I5) -> Dot Product2/1
  Dot Product1/1 -> Dot Product2/2, Dot Product9/1
  Trigonometric Function/1 -> Dot Product1/1, Dot Product3/1
  Dot Product3/1 -> Dot Product7/2
  Dot Product4/1 -> Dot Product8/1, Dot Product10/1
  Dot Product13/1 -> Sum2/2
  Dot Product2/1 -> Sum/1
  Dot Product6/1 -> Sum/2
  Dot Product7/1 -> Sum/3
  Dot Product8/1 -> Sum/4
  Dot Product9/1 -> Sum/5
  Dot Product10/1 -> Sum/6
  Dot Product11/1 -> Sum/7
  Sum2/1 -> Gain1/1
  Gain1/1 -> c31/1

== system PUMA_fuzzy_t1/3-Link PUMA Robot-Block /K or I matrix = fct (tau: torque, B, C, G, dteta) /C matrix/c32 ==
  teta3 : Inport
  Dot Product1 : DotProduct  InputSameDT=on  OutDataTypeStr=Inherit: Inherit via internal rule
  Dot Product2 : DotProduct  InputSameDT=on  OutDataTypeStr=Inherit: Inherit via internal rule
  Dot Product3 : DotProduct  InputSameDT=on  OutDataTypeStr=Inherit: Inherit via internal rule
  Gain1 : Gain  Gain=-1
  I12 : Subsystem
  I16 : Subsystem
  I5 : Subsystem
  SinCos(teta2+teta3) : aerolibutil/SinCos
      settings: SourceProductName=Aerospace Blockset  SourceProductBaseCode=AE
  Sum2 : Sum  Inputs=|-++
  c32 : Outport
  wires:
  teta3/1 -> SinCos(teta2+teta3)/1
  Dot Product3/1 -> Sum2/1
  Dot Product1/1 -> Sum2/2
  Dot Product2/1 -> Sum2/3
  I12/1(I12) -> Dot Product3/1
  I5/1(I5) -> Dot Product1/2
  I16/1(I16) -> Dot Product2/2
  SinCos(teta2+teta3)/2 -> Dot Product2/1, Dot Product1/1
  SinCos(teta2+teta3)/1 -> Dot Product3/2
  Sum2/1 -> Gain1/1
  Gain1/1 -> c32/1

== system PUMA_fuzzy_t1/3-Link PUMA Robot-Block /K or I matrix = fct (tau: torque, B, C, G, dteta) /C matrix/c51 ==
  teta2 : Inport
  teta3 : Inport  Port=2
  Dot Product{,1..5} (6 alike) : DotProduct  InputSameDT=on  OutDataTypeStr=Inherit: Inherit via internal rule
  Gain : Gain  Gain=-1
  Gain1 : Gain  Gain=-1
  I15 : Subsystem
  I16 : Subsystem
  I22 : Subsystem
  SinCos(teta2+teta3) : aerolibutil/SinCos
      settings: SourceProductName=Aerospace Blockset  SourceProductBaseCode=AE
  Sum2 : Sum  Inputs=|++++
  Sum3 : Sum  Inputs=|++
  Trigonometric Function : Trigonometry  Operator=cos
  c51 : Outport
  wires:
  teta2/1 -> Sum3/1, Trigonometric Function/1
  teta3/1 -> Sum3/2
  Sum3/1 -> SinCos(teta2+teta3)/1
  SinCos(teta2+teta3)/1 -> Dot Product/1
  SinCos(teta2+teta3)/2 -> Dot Product/2, Dot Product3/1, Dot Product5/1, Dot Product5/2
  Dot Product/1 -> Gain1/1, Dot Product1/1
  I15/1(I15) -> Dot Product1/2
  I16/1(I16) -> Dot Product2/2
  Dot Product3/1 -> Dot Product2/1
  Trigonometric Function/1 -> Dot Product3/2
  Sum2/1 -> Gain/1
  Gain/1 -> c51/1
  I22/1(I22) -> Dot Product4/2
  Dot Product5/1 -> Dot Product4/1
  Gain1/1 -> Sum2/1
  Dot Product1/1 -> Sum2/2
  Dot Product2/1 -> Sum2/3
  Dot Product4/1 -> Sum2/4

== system PUMA_fuzzy_t1/3-Link PUMA Robot-Block /K or I matrix = fct (tau: torque, B, C, G, dteta) /C matrix/c52 ==
  teta3 : Inport
  Dot Product2 : DotProduct  InputSameDT=on  OutDataTypeStr=Inherit: Inherit via internal rule
  Gain : Gain  Gain=-1
  I16 : Subsystem
  I22 : Subsystem
  Sum2 : Sum  Inputs=|++
  cos(teta3) : Trigonometry  Operator=cos
  c52 : Outport
  wires:
  teta3/1 -> cos(teta3)/1
  Sum2/1 -> Gain/1
  Gain/1 -> c52/1
  Dot Product2/1 -> Sum2/1
  I22/1(I22) -> Sum2/2
  I16/1(I16) -> Dot Product2/1
  cos(teta3)/1 -> Dot Product2/2

== system PUMA_fuzzy_t1/3-Link PUMA Robot-Block /K or I matrix = fct (tau: torque, B, C, G, dteta) /Gravity matrix/g2 term ==
  teta2 : Inport
  teta3 : Inport  Port=2
  Dot Product{,1..4} (5 alike) : DotProduct  InputSameDT=on  OutDataTypeStr=Inherit: Inherit via internal rule
  Sum : Sum  Inputs=|++
  Sum4 : Sum  Inputs=|+++++
  cos(teta2) : Trigonometry  Operator=cos
  cos(teta2+teta3) : Trigonometry  Operator=cos
  g1 : Subsystem
  g2 : Subsystem
  g3 : Subsystem
  g4 : Subsystem
  g5 : Subsystem
  sin(teta2) : Trigonometry
  sin(teta2+teta3) : Trigonometry
  G2 : Outport
  wires:
  teta2/1 -> Sum/1, cos(teta2)/1, sin(teta2)/1
  teta3/1 -> Sum/2
  Sum/1 -> sin(teta2+teta3)/1, cos(teta2+teta3)/1
  g1/1(g1) -> Dot Product/1
  cos(teta2)/1 -> Dot Product/2
  sin(teta2+teta3)/1 -> Dot Product1/1, Dot Product4/1
  g2/1(g2) -> Dot Product1/2
  sin(teta2)/1 -> Dot Product2/1
  g3/1(g3) -> Dot Product2/2
  g4/1(g4) -> Dot Product3/2
  cos(teta2+teta3)/1 -> Dot Product3/1
  g5/1(g5) -> Dot Product4/2
  Dot Product/1 -> Sum4/1
  Dot Product2/1 -> Sum4/2
  Dot Product1/1 -> Sum4/3
  Dot Product3/1 -> Sum4/4
  Dot Product4/1 -> Sum4/5
  Sum4/1 -> G2/1

== system PUMA_fuzzy_t1/3-Link PUMA Robot-Block /K or I matrix = fct (tau: torque, B, C, G, dteta) /Gravity matrix/g3 term ==
  teta2 : Inport
  teta3 : Inport  Port=2
  Dot Product5 : DotProduct  InputSameDT=on  OutDataTypeStr=Inherit: Inherit via internal rule
  Dot Product6 : DotProduct  InputSameDT=on  OutDataTypeStr=Inherit: Inherit via internal rule
  Dot Product7 : DotProduct  InputSameDT=on  OutDataTypeStr=Inherit: Inherit via internal rule
  Sum5 : Sum  Inputs=|++
  Sum6 : Sum  Inputs=|+++
  cos(teta2+teta3) : Trigonometry  Operator=cos
  g2 : Subsystem
  g4 : Subsystem
  g5 : Subsystem
  sin(teta2+teta3) : Trigonometry
  G3 : Outport
  wires:
  teta2/1 -> Sum5/1
  teta3/1 -> Sum5/2
  Sum5/1 -> sin(teta2+teta3)/1, cos(teta2+teta3)/1
  Dot Product5/1 -> Sum6/1
  Dot Product7/1 -> Sum6/2
  Dot Product6/1 -> Sum6/3
  Sum6/1 -> G3/1
  sin(teta2+teta3)/1 -> Dot Product5/2, Dot Product6/1
  g2/1(g2) -> Dot Product5/1
  cos(teta2+teta3)/1 -> Dot Product7/1
  g4/1(g4) -> Dot Product7/2
  g5/1(g5) -> Dot Product6/2

== system PUMA_fuzzy_t1/3-Link PUMA Robot-Block /K or I matrix = fct (tau: torque, B, C, G, dteta) /Gravity matrix/g5 term ==
  teta2 : Inport
  teta3 : Inport  Port=2
  Dot Product6 : DotProduct  InputSameDT=on  OutDataTypeStr=Inherit: Inherit via internal rule
  Sum5 : Sum  Inputs=|++
  g5 : Subsystem
  sin(teta2+teta3) : Trigonometry
  G5 : Outport
  wires:
  teta2/1 -> Sum5/1
  teta3/1 -> Sum5/2
  Sum5/1 -> sin(teta2+teta3)/1
  sin(teta2+teta3)/1 -> Dot Product6/1
  g5/1(g5) -> Dot Product6/2
  Dot Product6/1 -> G5/1

== system PUMA_fuzzy_t1/3-Link PUMA Robot-Block /K or I matrix = fct (tau: torque, B, C, G, dteta) /B matrix/b112/I10 ==
  AI10 actual I10 : Constant  Value=-0.0213
  Sum4 : Sum  Inputs=|++
  UI10 uncertainty added to I10 +- 0.022 max : Constant  Value=UI10
  I10 : Outport
  wires:
  AI10 actual I10/1 -> Sum4/1
  UI10 uncertainty added to I10 +- 0.022 max/1 -> Sum4/2
  Sum4/1 -> I10/1

== system PUMA_fuzzy_t1/3-Link PUMA Robot-Block /K or I matrix = fct (tau: torque, B, C, G, dteta) /B matrix/b112/I11 ==
  AI11 actual I11 : Constant  Value=-0.0142
  Sum4 : Sum  Inputs=|++
  UI11 uncertainty added to I11 +- 0.007 max : Constant  Value=UI11
  I11 : Outport
  wires:
  AI11 actual I11/1 -> Sum4/1
  UI11 uncertainty added to I11 +- 0.007 max/1 -> Sum4/2
  Sum4/1 -> I11/1

== system PUMA_fuzzy_t1/3-Link PUMA Robot-Block /K or I matrix = fct (tau: torque, B, C, G, dteta) /B matrix/b112/I12 ==
  AI12 actual I12 : Constant  Value=-0.011
  Sum4 : Sum  Inputs=|++
  UI12 uncertainty added to I12 +- 0.0011 max : Constant  Value=UI12
  I12 : Outport
  wires:
  AI12 actual I12/1 -> Sum4/1
  UI12 uncertainty added to I12 +- 0.0011 max/1 -> Sum4/2
  Sum4/1 -> I12/1

== system PUMA_fuzzy_t1/3-Link PUMA Robot-Block /K or I matrix = fct (tau: torque, B, C, G, dteta) /B matrix/b112/I15 ==
  AI15 actual I15 : Constant  Value=0.00125
  Sum4 : Sum  Inputs=|++
  UI15 uncertainty added to I15 +- 0.0003 max : Constant  Value=UI15
  I15 : Outport
  wires:
  AI15 actual I15/1 -> Sum4/1
  UI15 uncertainty added to I15 +- 0.0003 max/1 -> Sum4/2
  Sum4/1 -> I15/1

== system PUMA_fuzzy_t1/3-Link PUMA Robot-Block /K or I matrix = fct (tau: torque, B, C, G, dteta) /B matrix/b112/I16 ==
  AI16 actual I16 : Constant  Value=0.00124
  Sum4 : Sum  Inputs=|++
  UI16 uncertainty added to I16 +- 0.0003 max : Constant  Value=UI16
  I16 : Outport
  wires:
  AI16 actual I16/1 -> Sum4/1
  UI16 uncertainty added to I16 +- 0.0003 max/1 -> Sum4/2
  Sum4/1 -> I16/1

== system PUMA_fuzzy_t1/3-Link PUMA Robot-Block /K or I matrix = fct (tau: torque, B, C, G, dteta) /B matrix/b112/I21 ==
  AI21 actual I21 : Constant  Value=-0.0001
  Sum4 : Sum  Inputs=|++
  UI21 uncertainty added to I21 +- 0.0006 max : Constant  Value=UI21
  I21 : Outport
  wires:
  AI21 actual I21/1 -> Sum4/1
  UI21 uncertainty added to I21 +- 0.0006 max/1 -> Sum4/2
  Sum4/1 -> I21/1

== system PUMA_fuzzy_t1/3-Link PUMA Robot-Block /K or I matrix = fct (tau: torque, B, C, G, dteta) /B matrix/b112/I22 ==
  AI22 actual I22 : Constant  Value=-0.000058
  Sum4 : Sum  Inputs=|++
  UI22 uncertainty added to I22 +- 0.000015 max : Constant  Value=UI22
  I22 : Outport
  wires:
  AI22 actual I22/1 -> Sum4/1
  UI22 uncertainty added to I22 +- 0.000015 max/1 -> Sum4/2
  Sum4/1 -> I22/1

== system PUMA_fuzzy_t1/3-Link PUMA Robot-Block /K or I matrix = fct (tau: torque, B, C, G, dteta) /B matrix/b112/I3 ==
  AI3 actual I3 : Constant  Value=1.38
  Sum4 : Sum  Inputs=|++
  UI3 uncertainty added to I3 +- 0.05 max : Constant  Value=UI3
  I3 : Outport
  wires:
  AI3 actual I3/1 -> Sum4/1
  UI3 uncertainty added to I3 +- 0.05 max/1 -> Sum4/2
  Sum4/1 -> I3/1

== system PUMA_fuzzy_t1/3-Link PUMA Robot-Block /K or I matrix = fct (tau: torque, B, C, G, dteta) /B matrix/b112/I5 ==
  AI5 actual I5 : Constant  Value=0.372
  Sum4 : Sum  Inputs=|++
  UI5 uncertainty added to I5 +- 0.05 max : Constant  Value=UI5
  I5 : Outport
  wires:
  AI5 actual I5/1 -> Sum4/1
  UI5 uncertainty added to I5 +- 0.05 max/1 -> Sum4/2
  Sum4/1 -> I5/1

== system PUMA_fuzzy_t1/3-Link PUMA Robot-Block /K or I matrix = fct (tau: torque, B, C, G, dteta) /B matrix/b112/I7 ==
  AI7 actual I7 : Constant  Value=0.298
  Sum4 : Sum  Inputs=|++
  UI7 uncertainty added to I7 +- 0.029 max : Constant  Value=UI7
  I7 : Outport
  wires:
  AI7 actual I7/1 -> Sum4/1
  UI7 uncertainty added to I7 +- 0.029 max/1 -> Sum4/2
  Sum4/1 -> I7/1

== system PUMA_fuzzy_t1/3-Link PUMA Robot-Block /K or I matrix = fct (tau: torque, B, C, G, dteta) /B matrix/b113/I10 ==
  AI10 actual I10 : Constant  Value=-0.0213
  Sum4 : Sum  Inputs=|++
  UI10 uncertainty added to I10 +- 0.022 max : Constant  Value=UI10
  I10 : Outport
  wires:
  AI10 actual I10/1 -> Sum4/1
  UI10 uncertainty added to I10 +- 0.022 max/1 -> Sum4/2
  Sum4/1 -> I10/1

== system PUMA_fuzzy_t1/3-Link PUMA Robot-Block /K or I matrix = fct (tau: torque, B, C, G, dteta) /B matrix/b113/I12 ==
  AI12 actual I12 : Constant  Value=-0.011
  Sum4 : Sum  Inputs=|++
  UI12 uncertainty added to I12 +- 0.0011 max : Constant  Value=UI12
  I12 : Outport
  wires:
  AI12 actual I12/1 -> Sum4/1
  UI12 uncertainty added to I12 +- 0.0011 max/1 -> Sum4/2
  Sum4/1 -> I12/1

== system PUMA_fuzzy_t1/3-Link PUMA Robot-Block /K or I matrix = fct (tau: torque, B, C, G, dteta) /B matrix/b113/I15 ==
  AI15 actual I15 : Constant  Value=0.00125
  Sum4 : Sum  Inputs=|++
  UI15 uncertainty added to I15 +- 0.0003 max : Constant  Value=UI15
  I15 : Outport
  wires:
  AI15 actual I15/1 -> Sum4/1
  UI15 uncertainty added to I15 +- 0.0003 max/1 -> Sum4/2
  Sum4/1 -> I15/1

== system PUMA_fuzzy_t1/3-Link PUMA Robot-Block /K or I matrix = fct (tau: torque, B, C, G, dteta) /B matrix/b113/I16 ==
  AI16 actual I16 : Constant  Value=0.00124
  Sum4 : Sum  Inputs=|++
  UI16 uncertainty added to I16 +- 0.0003 max : Constant  Value=UI16
  I16 : Outport
  wires:
  AI16 actual I16/1 -> Sum4/1
  UI16 uncertainty added to I16 +- 0.0003 max/1 -> Sum4/2
  Sum4/1 -> I16/1

== system PUMA_fuzzy_t1/3-Link PUMA Robot-Block /K or I matrix = fct (tau: torque, B, C, G, dteta) /B matrix/b113/I21 ==
  AI21 actual I21 : Constant  Value=-0.0001
  Sum4 : Sum  Inputs=|++
  UI21 uncertainty added to I21 +- 0.0006 max : Constant  Value=UI21
  I21 : Outport
  wires:
  AI21 actual I21/1 -> Sum4/1
  UI21 uncertainty added to I21 +- 0.0006 max/1 -> Sum4/2
  Sum4/1 -> I21/1

== system PUMA_fuzzy_t1/3-Link PUMA Robot-Block /K or I matrix = fct (tau: torque, B, C, G, dteta) /B matrix/b113/I22 ==
  AI22 actual I22 : Constant  Value=-0.000058
  Sum4 : Sum  Inputs=|++
  UI22 uncertainty added to I22 +- 0.000015 max : Constant  Value=UI22
  I22 : Outport
  wires:
  AI22 actual I22/1 -> Sum4/1
  UI22 uncertainty added to I22 +- 0.000015 max/1 -> Sum4/2
  Sum4/1 -> I22/1

== system PUMA_fuzzy_t1/3-Link PUMA Robot-Block /K or I matrix = fct (tau: torque, B, C, G, dteta) /B matrix/b113/I5 ==
  AI5 actual I5 : Constant  Value=0.372
  Sum4 : Sum  Inputs=|++
  UI5 uncertainty added to I5 +- 0.05 max : Constant  Value=UI5
  I5 : Outport
  wires:
  AI5 actual I5/1 -> Sum4/1
  UI5 uncertainty added to I5 +- 0.05 max/1 -> Sum4/2
  Sum4/1 -> I5/1

== system PUMA_fuzzy_t1/3-Link PUMA Robot-Block /K or I matrix = fct (tau: torque, B, C, G, dteta) /B matrix/b113/I7 ==
  AI7 actual I7 : Constant  Value=0.298
  Sum4 : Sum  Inputs=|++
  UI7 uncertainty added to I7 +- 0.029 max : Constant  Value=UI7
  I7 : Outport
  wires:
  AI7 actual I7/1 -> Sum4/1
  UI7 uncertainty added to I7 +- 0.029 max/1 -> Sum4/2
  Sum4/1 -> I7/1

== system PUMA_fuzzy_t1/3-Link PUMA Robot-Block /K or I matrix = fct (tau: torque, B, C, G, dteta) /B matrix/b115/I15 ==
  AI15 actual I15 : Constant  Value=0.00125
  Sum4 : Sum  Inputs=|++
  UI15 uncertainty added to I15 +- 0.0003 max : Constant  Value=UI15
  I15 : Outport
  wires:
  AI15 actual I15/1 -> Sum4/1
  UI15 uncertainty added to I15 +- 0.0003 max/1 -> Sum4/2
  Sum4/1 -> I15/1

== system PUMA_fuzzy_t1/3-Link PUMA Robot-Block /K or I matrix = fct (tau: torque, B, C, G, dteta) /B matrix/b115/I16 ==
  AI16 actual I16 : Constant  Value=0.00124
  Sum4 : Sum  Inputs=|++
  UI16 uncertainty added to I16 +- 0.0003 max : Constant  Value=UI16
  I16 : Outport
  wires:
  AI16 actual I16/1 -> Sum4/1
  UI16 uncertainty added to I16 +- 0.0003 max/1 -> Sum4/2
  Sum4/1 -> I16/1

== system PUMA_fuzzy_t1/3-Link PUMA Robot-Block /K or I matrix = fct (tau: torque, B, C, G, dteta) /B matrix/b115/I22 ==
  AI22 actual I22 : Constant  Value=-0.000058
  Sum4 : Sum  Inputs=|++
  UI22 uncertainty added to I22 +- 0.000015 max : Constant  Value=UI22
  I22 : Outport
  wires:
  AI22 actual I22/1 -> Sum4/1
  UI22 uncertainty added to I22 +- 0.000015 max/1 -> Sum4/2
  Sum4/1 -> I22/1

== system PUMA_fuzzy_t1/3-Link PUMA Robot-Block /K or I matrix = fct (tau: torque, B, C, G, dteta) /B matrix/b123/I13 ==
  AI13 actual I13 : Constant  Value=-0.00379
  Sum4 : Sum  Inputs=|++
  UI13 uncertainty added to I13 +- 0.0009 max : Constant  Value=UI13
  I13 : Outport
  wires:
  AI13 actual I13/1 -> Sum4/1
  UI13 uncertainty added to I13 +- 0.0009 max/1 -> Sum4/2
  Sum4/1 -> I13/1

== system PUMA_fuzzy_t1/3-Link PUMA Robot-Block /K or I matrix = fct (tau: torque, B, C, G, dteta) /B matrix/b123/I18 ==
  AI18 actual I18 : Constant  Value=0.000431
  Sum4 : Sum  Inputs=|++
  UI18 uncertainty added to I18 +- 0.0003 max : Constant  Value=UI18
  I18 : Outport
  wires:
  AI18 actual I18/1 -> Sum4/1
  UI18 uncertainty added to I18 +- 0.0003 max/1 -> Sum4/2
  Sum4/1 -> I18/1

== system PUMA_fuzzy_t1/3-Link PUMA Robot-Block /K or I matrix = fct (tau: torque, B, C, G, dteta) /B matrix/b123/I8 ==
  AI8 actual I8 : Constant  Value=-0.134
  Sum4 : Sum  Inputs=|++
  UI8 uncertainty added to I8 +- 0.014 max : Constant  Value=UI8
  I8 : Outport
  wires:
  AI8 actual I8/1 -> Sum4/1
  UI8 uncertainty added to I8 +- 0.014 max/1 -> Sum4/2
  Sum4/1 -> I8/1

== system PUMA_fuzzy_t1/3-Link PUMA Robot-Block /K or I matrix = fct (tau: torque, B, C, G, dteta) /B matrix/b214/I14 ==
  AI14 actual I14 : Constant  Value=0.00164
  Sum4 : Sum  Inputs=|++
  UI14 uncertainty added to I14 +- 0.0009 max : Constant  Value=UI14
  I14 : Outport
  wires:
  AI14 actual I14/1 -> Sum4/1
  UI14 uncertainty added to I14 +- 0.0009 max/1 -> Sum4/2
  Sum4/1 -> I14/1

== system PUMA_fuzzy_t1/3-Link PUMA Robot-Block /K or I matrix = fct (tau: torque, B, C, G, dteta) /B matrix/b214/I19 ==
  AI19 actual I19 : Constant  Value=0.0003
  Sum4 : Sum  Inputs=|++
  UI19 uncertainty added to I19 +- 0.0003 max : Constant  Value=UI19
  I19 : Outport
  wires:
  AI19 actual I19/1 -> Sum4/1
  UI19 uncertainty added to I19 +- 0.0003 max/1 -> Sum4/2
  Sum4/1 -> I19/1

== system PUMA_fuzzy_t1/3-Link PUMA Robot-Block /K or I matrix = fct (tau: torque, B, C, G, dteta) /B matrix/b214/I20 ==
  AI20 actual I20 : Constant  Value=-0.000202
  Sum4 : Sum  Inputs=|++
  UI20 uncertainty added to I20 +- 0.0008 max : Constant  Value=UI20
  I20 : Outport
  wires:
  AI20 actual I20/1 -> Sum4/1
  UI20 uncertainty added to I20 +- 0.0008 max/1 -> Sum4/2
  Sum4/1 -> I20/1

== system PUMA_fuzzy_t1/3-Link PUMA Robot-Block /K or I matrix = fct (tau: torque, B, C, G, dteta) /B matrix/b223/I12 ==
  AI12 actual I12 : Constant  Value=-0.011
  Sum4 : Sum  Inputs=|++
  UI12 uncertainty added to I12 +- 0.0011 max : Constant  Value=UI12
  I12 : Outport
  wires:
  AI12 actual I12/1 -> Sum4/1
  UI12 uncertainty added to I12 +- 0.0011 max/1 -> Sum4/2
  Sum4/1 -> I12/1

== system PUMA_fuzzy_t1/3-Link PUMA Robot-Block /K or I matrix = fct (tau: torque, B, C, G, dteta) /B matrix/b223/I16 ==
  AI16 actual I16 : Constant  Value=0.00124
  Sum4 : Sum  Inputs=|++
  UI16 uncertainty added to I16 +- 0.0003 max : Constant  Value=UI16
  I16 : Outport
  wires:
  AI16 actual I16/1 -> Sum4/1
  UI16 uncertainty added to I16 +- 0.0003 max/1 -> Sum4/2
  Sum4/1 -> I16/1

== system PUMA_fuzzy_t1/3-Link PUMA Robot-Block /K or I matrix = fct (tau: torque, B, C, G, dteta) /B matrix/b223/I5 ==
  AI5 actual I5 : Constant  Value=0.372
  Sum4 : Sum  Inputs=|++
  UI5 uncertainty added to I5 +- 0.05 max : Constant  Value=UI5
  I5 : Outport
  wires:
  AI5 actual I5/1 -> Sum4/1
  UI5 uncertainty added to I5 +- 0.05 max/1 -> Sum4/2
  Sum4/1 -> I5/1

== system PUMA_fuzzy_t1/3-Link PUMA Robot-Block /K or I matrix = fct (tau: torque, B, C, G, dteta) /B matrix/b225/I16 ==
  AI16 actual I16 : Constant  Value=0.00124
  Sum4 : Sum  Inputs=|++
  UI16 uncertainty added to I16 +- 0.0003 max : Constant  Value=UI16
  I16 : Outport
  wires:
  AI16 actual I16/1 -> Sum4/1
  UI16 uncertainty added to I16 +- 0.0003 max/1 -> Sum4/2
  Sum4/1 -> I16/1

== system PUMA_fuzzy_t1/3-Link PUMA Robot-Block /K or I matrix = fct (tau: torque, B, C, G, dteta) /B matrix/b225/I22 ==
  AI22 actual I22 : Constant  Value=-0.000058
  Sum4 : Sum  Inputs=|++
  UI22 uncertainty added to I22 +- 0.000015 max : Constant  Value=UI22
  I22 : Outport
  wires:
  AI22 actual I22/1 -> Sum4/1
  UI22 uncertainty added to I22 +- 0.000015 max/1 -> Sum4/2
  Sum4/1 -> I22/1

== system PUMA_fuzzy_t1/3-Link PUMA Robot-Block /K or I matrix = fct (tau: torque, B, C, G, dteta) /B matrix/b235/I16 ==
  AI16 actual I16 : Constant  Value=0.00124
  Sum4 : Sum  Inputs=|++
  UI16 uncertainty added to I16 +- 0.0003 max : Constant  Value=UI16
  I16 : Outport
  wires:
  AI16 actual I16/1 -> Sum4/1
  UI16 uncertainty added to I16 +- 0.0003 max/1 -> Sum4/2
  Sum4/1 -> I16/1

== system PUMA_fuzzy_t1/3-Link PUMA Robot-Block /K or I matrix = fct (tau: torque, B, C, G, dteta) /B matrix/b235/I22 ==
  AI22 actual I22 : Constant  Value=-0.000058
  Sum4 : Sum  Inputs=|++
  UI22 uncertainty added to I22 +- 0.000015 max : Constant  Value=UI22
  I22 : Outport
  wires:
  AI22 actual I22/1 -> Sum4/1
  UI22 uncertainty added to I22 +- 0.000015 max/1 -> Sum4/2
  Sum4/1 -> I22/1

== system PUMA_fuzzy_t1/3-Link PUMA Robot-Block /K or I matrix = fct (tau: torque, B, C, G, dteta) /B matrix/b314/I14 ==
  AI14 actual I14 : Constant  Value=0.00164
  Sum4 : Sum  Inputs=|++
  UI14 uncertainty added to I14 +- 0.0009 max : Constant  Value=UI14
  I14 : Outport
  wires:
  AI14 actual I14/1 -> Sum4/1
  UI14 uncertainty added to I14 +- 0.0009 max/1 -> Sum4/2
  Sum4/1 -> I14/1

== system PUMA_fuzzy_t1/3-Link PUMA Robot-Block /K or I matrix = fct (tau: torque, B, C, G, dteta) /B matrix/b314/I19 ==
  AI19 actual I19 : Constant  Value=0.0003
  Sum4 : Sum  Inputs=|++
  UI19 uncertainty added to I19 +- 0.0003 max : Constant  Value=UI19
  I19 : Outport
  wires:
  AI19 actual I19/1 -> Sum4/1
  UI19 uncertainty added to I19 +- 0.0003 max/1 -> Sum4/2
  Sum4/1 -> I19/1

== system PUMA_fuzzy_t1/3-Link PUMA Robot-Block /K or I matrix = fct (tau: torque, B, C, G, dteta) /B matrix/b314/I20 ==
  AI20 actual I20 : Constant  Value=-0.000202
  Sum4 : Sum  Inputs=|++
  UI20 uncertainty added to I20 +- 0.0008 max : Constant  Value=UI20
  I20 : Outport
  wires:
  AI20 actual I20/1 -> Sum4/1
  UI20 uncertainty added to I20 +- 0.0008 max/1 -> Sum4/2
  Sum4/1 -> I20/1

== system PUMA_fuzzy_t1/3-Link PUMA Robot-Block /K or I matrix = fct (tau: torque, B, C, G, dteta) /B matrix/b412/I14 ==
  AI14 actual I14 : Constant  Value=0.00164
  Sum4 : Sum  Inputs=|++
  UI14 uncertainty added to I14 +- 0.0009 max : Constant  Value=UI14
  I14 : Outport
  wires:
  AI14 actual I14/1 -> Sum4/1
  UI14 uncertainty added to I14 +- 0.0009 max/1 -> Sum4/2
  Sum4/1 -> I14/1
